simulink model "Modell_4"  (R2017b)
settings: Solver=ode45  StartTime=0.0  StopTime=1  MaxStep=1e-4  RelTol=1e-3
settings Model: Creator=lukasschwoerer  LastModifiedBy=lukasschwoerer

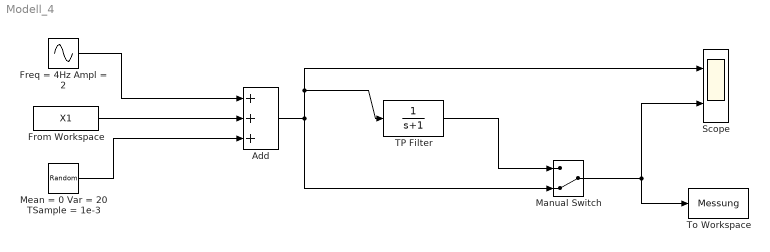
== system Modell_4 ==
  Add : Sum  Inputs=+++
  Freq = 4Hz Ampl = 2 : Sin  Amplitude=2  Frequency=2*pi*4  SampleTime=0
  From Workspace : FromWorkspace  VariableName=X1  SampleTime=0
  Manual Switch : ManualSwitch  CurrentSetting=0
  Mean = 0 Var = 20 TSample = 1e-3 : RandomNumber  Variance=20  SampleTime=1e-3
  Scope : Scope  NumInputPorts=2
  "TP Filter " : TransferFcn  Denominator=[1 1]
  To Workspace : ToWorkspace  VariableName=Messung  SaveFormat=Structure With Time  SampleTime=-1
  wires:
  Freq = 4Hz Ampl = 2/1 -> Add/1
  From Workspace/1 -> Add/2
  Mean = 0 Var = 20 TSample = 1e-3/1 -> Add/3
  Add/1 -> "TP Filter "/1, Scope/1, Manual Switch/2
  "TP Filter "/1 -> Manual Switch/1
  Manual Switch/1 -> To Workspace/1, Scope/2
